simulink model "dinamica_formacao_voo"  (R2025a)
settings: Solver=ode15s  StartTime=0.0  StopTime=1424.2163  MaxStep=0.001*T  RelTol=1e-3
values from neighbouring files (symbols this model uses):
  a0 = 8e6    (= 8000000)    [main_script.m]
  controle = true    [main_script.m]
  e0 = 0.1    [main_script.m]
  f0 = 0    [main_script.m]
  i = 0    [main_script.m]
  kx = 400    [main_script.m]
  ky = 200    [main_script.m]
  kz = 200    [main_script.m]
  lambdax = 1/(1e2)    (= 0.01)    [main_script.m]
  lambday = 1/(1e2)    (= 0.01)    [main_script.m]
  lambdaz = 1/(1e2)    (= 0.01)    [main_script.m]
  mi = 3.986004418e14    (= 398600441800000)    [main_script.m]
  Omega = 0    [main_script.m]
  phix = 30    [main_script.m]
  w0 = 0    [main_script.m]
  x0_controle = -0.01127*a0    (= -90160)    [main_script.m]
  x0_real = -0.0113*a0    (= -90400)    [main_script.m]
  x_dot0 = 0.02*sqrt(mi/a0^3)*a0    [main_script.m]
  y0 = 0*a0    (= 0)    [main_script.m]
  y_dot0 = 0.02*sqrt(mi/a0^3)*a0    [main_script.m]
  z0 = 0.1*a0    (= 800000)    [main_script.m]
  z_dot0 = 0*sqrt(mi/a0^3)*a0    [main_script.m]
settings Model: Creator=Erick_Tenorio

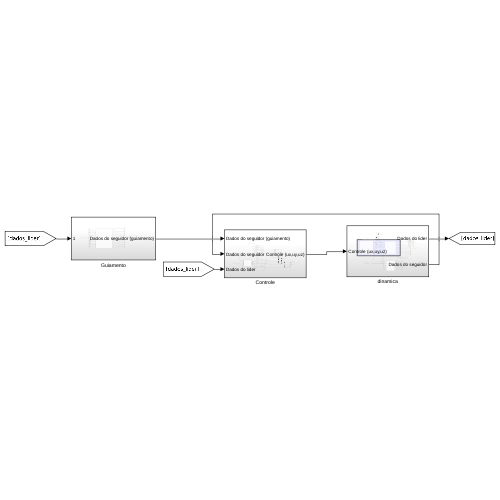
[thumbnail: Simulink's stored preview of the top-level diagram]
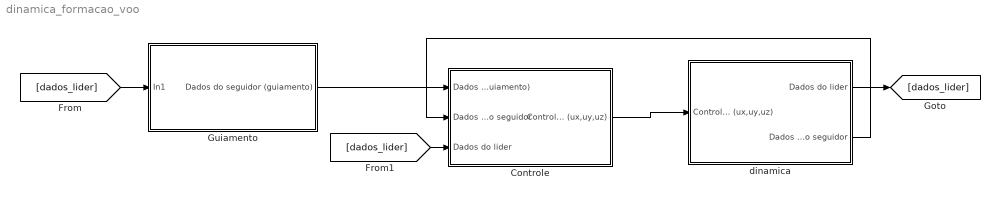
== system dinamica_formacao_voo ==
  Controle : Subsystem
  Guiamento : Subsystem
  dinamica : Subsystem
  wires:
  dinamica/1(Dados do lider) -> [dados_lider]
  [dados_lider] -> Guiamento/1(In1)
  Guiamento/1(Dados do seguidor (guiamento)) -> Controle/1(Dados do seguidor (guiamento))
  dinamica/2(Dados do seguidor) -> Controle/2(Dados do seguidor)
  [dados_lider] -> Controle/3(Dados do lider)
  Controle/1(Controle (ux,uy,uz)) -> dinamica/1(Controle (ux,uy,uz))

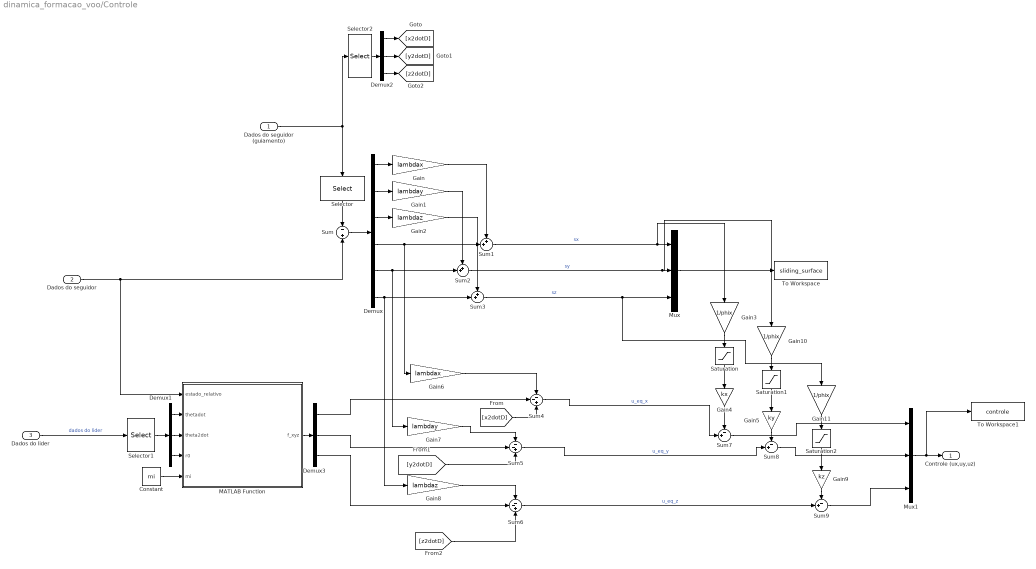
== system dinamica_formacao_voo/Controle ==
  Dados do seguidor (guiamento) : Inport
  Dados do seguidor : Inport  Port=2
  Dados do lider : Inport  Port=3
  Constant : Constant  Value=mi
  Demux : Demux  Outputs=6
  Demux1 : Demux  Outputs=3
  Demux2 : Demux  Outputs=3
  Demux3 : Demux  Outputs=3
  Gain : Gain  Gain=lambdax
  Gain1 : Gain  Gain=lambday
  Gain10 : Gain  Gain=1/phix
  Gain11 : Gain  Gain=1/phix
  Gain2 : Gain  Gain=lambdaz
  Gain3 : Gain  Gain=1/phix
  Gain4 : Gain  Gain=kx
  Gain5 : Gain  Gain=ky
  Gain6 : Gain  Gain=lambdax
  Gain7 : Gain  Gain=lambday
  Gain8 : Gain  Gain=lambdaz
  Gain9 : Gain  Gain=kz
  MATLAB Function : MATLAB Function  TreatAsAtomicUnit=on
  Mux : Mux  Inputs=3
  Mux1 : Mux  Inputs=3
  Saturation : Saturate  UpperLimit=1  LowerLimit=-1
  Saturation1 : Saturate  UpperLimit=1  LowerLimit=-1
  Saturation2 : Saturate  UpperLimit=1  LowerLimit=-1
  Selector : Selector  InputPortWidth=9  IndexOptions=Index vector (dialog)  Indices=[1 2 3 4 5 6]  OutputSizes=1
  Selector1 : Selector  InputPortWidth=7  IndexOptions=Index vector (dialog)  Indices=[3 4 1]  OutputSizes=1
  Selector2 : Selector  InputPortWidth=9  IndexOptions=Index vector (dialog)  Indices=[7 8 9]  OutputSizes=1
  Sum : Sum  Inputs=-|+
  Sum1 : Sum  Inputs=++|
  Sum2 : Sum  Inputs=++|
  Sum3 : Sum  Inputs=++|
  Sum4 : Sum  Inputs=--+
  Sum5 : Sum  Inputs=--+
  Sum6 : Sum  Inputs=--+
  Sum7 : Sum  Inputs=-+|
  Sum8 : Sum  Inputs=-+|
  Sum9 : Sum  Inputs=-+|
  To Workspace : ToWorkspace  VariableName=sliding_surface  SaveFormat=Timeseries  SampleTime=-1
  To Workspace1 : ToWorkspace  VariableName=controle  SaveFormat=Timeseries  SampleTime=-1
  Controle (ux,uy,uz) : Outport
  wires:
  Dados do seguidor (guiamento)/1 -> Selector2/1, Selector/1
  Dados do seguidor/1 -> Sum/2, MATLAB Function/1(estado_relativo)
  Sum/1 -> Demux/1
  Demux/1 -> Gain/1
  Demux/2 -> Gain1/1
  Demux/3 -> Gain2/1
  Gain/1 -> Sum1/1
  Demux/4 -> Gain6/1, Sum1/2
  Gain1/1 -> Sum2/1
  Demux/5 -> Gain7/1, Sum2/2
  Gain2/1 -> Sum3/1
  Demux/6 -> Gain8/1, Sum3/2
  Sum1/1 -> Mux/1, Gain3/1  "sx"
  Sum2/1 -> Gain10/1, Mux/2  "sy"
  Sum3/1 -> Gain11/1, Mux/3  "sz"
  Mux/1 -> To Workspace/1
  Dados do lider/1 -> Selector1/1  "dados do lider"
  Constant/1 -> MATLAB Function/5(mi)
  Selector/1 -> Sum/1
  Selector1/1 -> Demux1/1
  Demux1/1 -> MATLAB Function/2(thetadot)
  Demux1/2 -> MATLAB Function/3(theta2dot)
  Demux1/3 -> MATLAB Function/4(r0)
  Demux2/1 -> [x2dotD]
  Demux2/2 -> [y2dotD]
  Demux2/3 -> [z2dotD]
  Selector2/1 -> Demux2/1
  Gain6/1 -> Sum4/1
  Gain7/1 -> Sum5/1
  Gain8/1 -> Sum6/1
  [x2dotD] -> Sum4/3
  [y2dotD] -> Sum5/3
  [z2dotD] -> Sum6/3
  Sum5/1 -> Sum8/2  "u_eq_y"
  Sum6/1 -> Sum9/2  "u_eq_z"
  Sum4/1 -> Sum7/2  "u_eq_x"
  Gain3/1 -> Saturation/1
  Gain11/1 -> Saturation2/1
  Gain10/1 -> Saturation1/1
  Saturation/1 -> Gain4/1
  Saturation1/1 -> Gain5/1
  Saturation2/1 -> Gain9/1
  Gain9/1 -> Sum9/1
  Gain5/1 -> Sum8/1
  Gain4/1 -> Sum7/1
  Mux1/1 -> To Workspace1/1, Controle (ux,uy,uz)/1
  Sum7/1 -> Mux1/1
  Sum8/1 -> Mux1/2
  Sum9/1 -> Mux1/3
  MATLAB Function/1(f_xyz) -> Demux3/1
  Demux3/1 -> Sum4/2
  Demux3/2 -> Sum5/2
  Demux3/3 -> Sum6/2

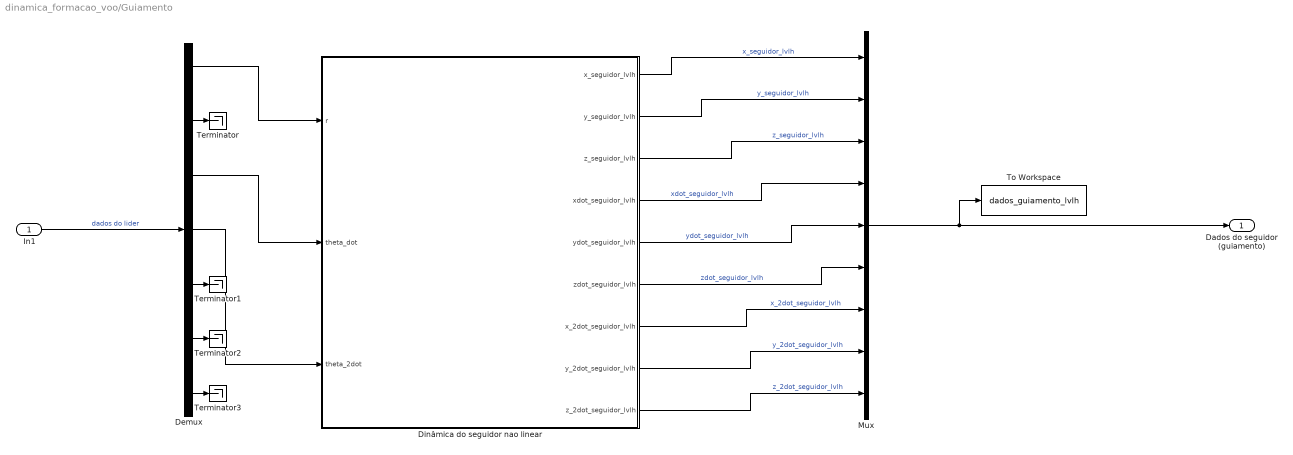
== system dinamica_formacao_voo/Guiamento ==
  In1 : Inport
  Demux : Demux  Outputs=7
  Dinâmica do seguidor nao linear : Subsystem
  Mux : Mux  Inputs=9
  Terminator{,1..3} (4 alike) : Terminator
  To Workspace : ToWorkspace  VariableName=dados_guiamento_lvlh  SaveFormat=Timeseries  SampleTime=-1
  Dados do seguidor (guiamento) : Outport
  wires:
  In1/1 -> Demux/1  "dados do lider"
  Dinâmica do seguidor nao linear/2(y_seguidor_lvlh) -> Mux/2  "y_seguidor_lvlh"
  Dinâmica do seguidor nao linear/3(z_seguidor_lvlh) -> Mux/3  "z_seguidor_lvlh"
  Dinâmica do seguidor nao linear/1(x_seguidor_lvlh) -> Mux/1  "x_seguidor_lvlh"
  Dinâmica do seguidor nao linear/4(xdot_seguidor_lvlh) -> Mux/4  "xdot_seguidor_lvlh"
  Dinâmica do seguidor nao linear/5(ydot_seguidor_lvlh) -> Mux/5  "ydot_seguidor_lvlh"
  Dinâmica do seguidor nao linear/6(zdot_seguidor_lvlh) -> Mux/6  "zdot_seguidor_lvlh"
  Mux/1 -> To Workspace/1, Dados do seguidor (guiamento)/1
  Demux/1 -> Dinâmica do seguidor nao linear/1(r)
  Demux/3 -> Dinâmica do seguidor nao linear/2(theta_dot)
  Demux/4 -> Dinâmica do seguidor nao linear/3(theta_2dot)
  Demux/2 -> Terminator/1
  Demux/5 -> Terminator1/1
  Demux/6 -> Terminator2/1
  Demux/7 -> Terminator3/1
  Dinâmica do seguidor nao linear/9(z_2dot_seguidor_lvlh) -> Mux/9  "z_2dot_seguidor_lvlh"
  Dinâmica do seguidor nao linear/8(y_2dot_seguidor_lvlh) -> Mux/8  "y_2dot_seguidor_lvlh"
  Dinâmica do seguidor nao linear/7(x_2dot_seguidor_lvlh) -> Mux/7  "x_2dot_seguidor_lvlh"

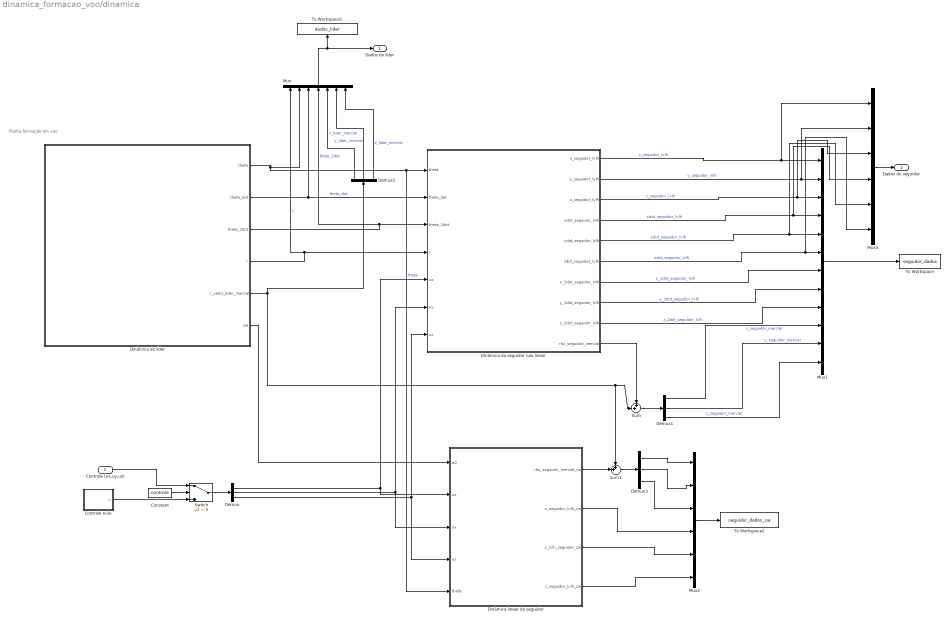
== system dinamica_formacao_voo/dinamica ==
  note: Planta formação em voo
  Controle (ux,uy,uz) : Inport
  Constant : Constant  Value=controle
  Controle nulo : Subsystem
  Demux{,1..3} (4 alike) : Demux  Outputs=3
  Dinâmica do líder : Subsystem
  Dinâmica do seguidor nao linear : Subsystem
  Dinâmica linear do seguidor : Subsystem
  Mux : Mux  Inputs=7
  Mux1 : Mux  Inputs=12
  Mux2 : Mux  Inputs=6
  Mux3 : Mux  Inputs=6
  Sum : Sum  Inputs=++|
  Sum1 : Sum  Inputs=++|
  Switch : Switch  Criteria=u2 > Threshold  SaturateOnIntegerOverflow=off  InputSameDT=off
  To Workspace : ToWorkspace  VariableName=seguidor_dados  SaveFormat=Timeseries  SampleTime=-1
  To Workspace1 : ToWorkspace  VariableName=dados_lider  SaveFormat=Timeseries  SampleTime=-1
  To Workspace2 : ToWorkspace  VariableName=seguidor_dados_cw  SaveFormat=Timeseries  SampleTime=-1
  Dados do lider : Outport
  Dados do seguidor : Outport  Port=2
  wires:
  Dinâmica do seguidor nao linear/7(x_2dot_seguidor_lvlh) -> Mux1/7  "x_2dot_seguidor_lvlh"
  Dinâmica do seguidor nao linear/10(rho_seguidor_inercial) -> Sum/1
  Demux2/3 -> Mux/7  "z_lider_inercial"
  Dinâmica do líder/5(r_vetor_lider_inercial) -> Sum1/1, Sum/2, Demux2/1
  Dinâmica do líder/6(a0) -> Dinâmica linear do seguidor/1(a0)
  Dinâmica do seguidor nao linear/5(ydot_seguidor_lvlh) -> Mux3/5, Mux1/5  "ydot_seguidor_lvlh"
  Demux1/3 -> Mux1/12  "z_seguidor_inercial"
  Demux/2 -> Dinâmica do seguidor nao linear/6(uy), Dinâmica linear do seguidor/3(uy)
  Demux3/3 -> Mux2/3
  Demux3/2 -> Mux2/2
  Demux1/2 -> Mux1/11  "y_seguidor_inercial"
  Dinâmica do seguidor nao linear/1(x_seguidor_lvlh) -> Mux3/1, Mux1/1  "x_seguidor_lvlh"
  Demux/1 -> Dinâmica do seguidor nao linear/5(ux), Dinâmica linear do seguidor/2(ux)
  Dinâmica do seguidor nao linear/9(z_2dot_seguidor_lvlh) -> Mux1/9  "z_2dot_seguidor_lvlh"
  Dinâmica do líder/3(theta_2dot) -> Mux/4, Dinâmica do seguidor nao linear/3(theta_2dot)  "theta_2dot"
  Mux/1 -> Dados do lider/1, To Workspace1/1
  Demux/3 -> Dinâmica do seguidor nao linear/7(uz), Dinâmica linear do seguidor/4(uz)
  Dinâmica do seguidor nao linear/8(y_2dot_seguidor_lvlh) -> Mux1/8  "y_2dot_seguidor_lvlh"
  Dinâmica do líder/4(r) -> Dinâmica do seguidor nao linear/4(r), Mux/1  "r"
  Dinâmica do seguidor nao linear/4(xdot_seguidor_lvlh) -> Mux3/4, Mux1/4  "xdot_seguidor_lvlh"
  Dinâmica do líder/1(theta) -> Dinâmica linear do seguidor/5(theta), Dinâmica do seguidor nao linear/1(theta), Mux/2  "theta"
  Mux1/1 -> To Workspace/1
  Demux2/1 -> Mux/5  "x_lider_inercial"
  Dinâmica do líder/2(theta_dot) -> Dinâmica do seguidor nao linear/2(theta_dot), Mux/3  "theta_dot"
  Demux2/2 -> Mux/6  "y_lider_inercial"
  Sum1/1 -> Demux3/1
  Dinâmica linear do seguidor/1(rho_seguidor_inercial_cw) -> Sum1/2
  Dinâmica do seguidor nao linear/6(zdot_seguidor_lvlh) -> Mux3/6, Mux1/6  "zdot_seguidor_lvlh"
  Dinâmica do seguidor nao linear/3(z_seguidor_lvlh) -> Mux3/3, Mux1/3  "z_seguidor_lvlh"
  Dinâmica do seguidor nao linear/2(y_seguidor_lvlh) -> Mux3/2, Mux1/2  "y_seguidor_lvlh"
  Sum/1 -> Demux1/1
  Demux1/1 -> Mux1/10  "x_seguidor_inercial"
  Dinâmica linear do seguidor/3(y_lvlh_seguidor_cw) -> Mux2/5
  Mux2/1 -> To Workspace2/1
  Dinâmica linear do seguidor/2(x_seguidor_lvlh_cw) -> Mux2/4
  Dinâmica linear do seguidor/4(z_seguidor_lvlh_cw) -> Mux2/6
  Demux3/1 -> Mux2/1
  Controle (ux,uy,uz)/1 -> Switch/1
  Controle nulo/1(u) -> Switch/3
  Switch/1 -> Demux/1
  Constant/1 -> Switch/2
  Mux3/1 -> Dados do seguidor/1

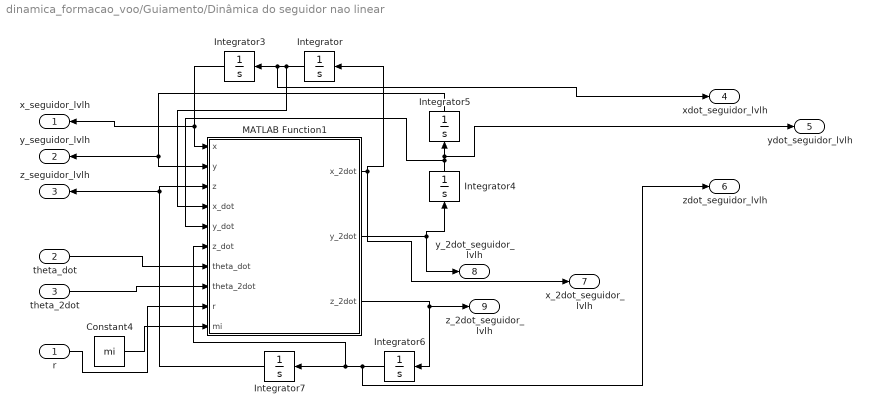
== system dinamica_formacao_voo/Guiamento/Dinâmica do seguidor nao linear ==
  r : Inport
  theta_dot : Inport  Port=2
  theta_2dot : Inport  Port=3
  Constant4 : Constant  Value=mi
  Integrator : Integrator  InitialCondition=x_dot0
  Integrator3 : Integrator  InitialCondition=x0_controle
  Integrator4 : Integrator  InitialCondition=y_dot0
  Integrator5 : Integrator  InitialCondition=y0
  Integrator6 : Integrator  InitialCondition=z_dot0
  Integrator7 : Integrator  InitialCondition=z0
  MATLAB Function1 : MATLAB Function  TreatAsAtomicUnit=on
  x_seguidor_lvlh : Outport
  y_seguidor_lvlh : Outport  Port=2
  z_seguidor_lvlh : Outport  Port=3
  xdot_seguidor_lvlh : Outport  Port=4
  ydot_seguidor_lvlh : Outport  Port=5
  zdot_seguidor_lvlh : Outport  Port=6
  x_2dot_seguidor_lvlh : Outport  Port=7
  y_2dot_seguidor_lvlh : Outport  Port=8
  z_2dot_seguidor_lvlh : Outport  Port=9
  wires:
  Integrator6/1 -> zdot_seguidor_lvlh/1, MATLAB Function1/6(z_dot), Integrator7/1
  Integrator/1 -> MATLAB Function1/4(x_dot), xdot_seguidor_lvlh/1, Integrator3/1
  MATLAB Function1/2(y_2dot) -> Integrator4/1, y_2dot_seguidor_lvlh/1
  Integrator5/1 -> MATLAB Function1/2(y), y_seguidor_lvlh/1
  MATLAB Function1/3(z_2dot) -> Integrator6/1, z_2dot_seguidor_lvlh/1
  Integrator3/1 -> MATLAB Function1/1(x), x_seguidor_lvlh/1
  Integrator4/1 -> MATLAB Function1/5(y_dot), ydot_seguidor_lvlh/1, Integrator5/1
  theta_dot/1 -> MATLAB Function1/7(theta_dot)
  Constant4/1 -> MATLAB Function1/10(mi)
  theta_2dot/1 -> MATLAB Function1/8(theta_2dot)
  MATLAB Function1/1(x_2dot) -> Integrator/1, x_2dot_seguidor_lvlh/1
  Integrator7/1 -> z_seguidor_lvlh/1, MATLAB Function1/3(z)
  r/1 -> MATLAB Function1/9(r)

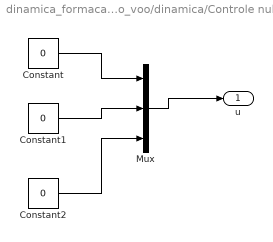
== system dinamica_formacao_voo/dinamica/Controle nulo ==
  Constant : Constant  Value=0
  Constant1 : Constant  Value=0
  Constant2 : Constant  Value=0
  Mux : Mux  Inputs=3
  u : Outport
  wires:
  Constant/1 -> Mux/1
  Constant1/1 -> Mux/2
  Constant2/1 -> Mux/3
  Mux/1 -> u/1

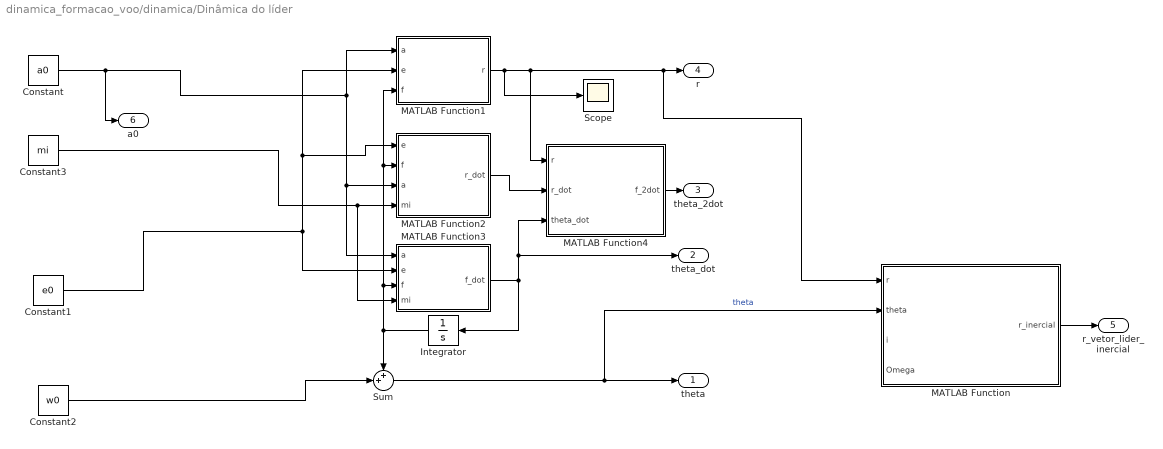
== system dinamica_formacao_voo/dinamica/Dinâmica do líder ==
  Constant : Constant  Value=a0
  Constant1 : Constant  Value=e0
  Constant2 : Constant  Value=w0
  Constant3 : Constant  Value=mi
  Integrator : Integrator  InitialCondition=f0
  MATLAB Function : MATLAB Function  TreatAsAtomicUnit=on
  MATLAB Function1 : MATLAB Function  TreatAsAtomicUnit=on
  MATLAB Function2 : MATLAB Function  TreatAsAtomicUnit=on
  MATLAB Function3 : MATLAB Function  TreatAsAtomicUnit=on
  MATLAB Function4 : MATLAB Function  TreatAsAtomicUnit=on
  Scope : Scope
      settings: ActiveDisplayYMinimum=7.0E+6  ActiveDisplayYMaximum=9.0E+6
  Sum : Sum  Inputs=++|
  theta : Outport
  theta_dot : Outport  Port=2
  theta_2dot : Outport  Port=3
  r : Outport  Port=4
  r_vetor_lider_inercial : Outport  Port=5
  a0 : Outport  Port=6
  wires:
  Constant/1 -> a0/1, MATLAB Function3/1(a), MATLAB Function2/3(a), MATLAB Function1/1(a)
  Constant1/1 -> MATLAB Function2/1(e), MATLAB Function1/2(e), MATLAB Function3/2(e)
  Constant2/1 -> Sum/2
  Constant3/1 -> MATLAB Function3/4(mi), MATLAB Function2/4(mi)
  MATLAB Function3/1(f_dot) -> theta_dot/1, MATLAB Function4/3(theta_dot), Integrator/1
  MATLAB Function1/1(r) -> Scope/1, MATLAB Function/1(r), r/1, MATLAB Function4/1(r)
  Integrator/1 -> Sum/1, MATLAB Function1/3(f), MATLAB Function2/2(f), MATLAB Function3/3(f)
  Sum/1 -> MATLAB Function/2(theta), theta/1  "theta"
  MATLAB Function2/1(r_dot) -> MATLAB Function4/2(r_dot)
  MATLAB Function4/1(f_2dot) -> theta_2dot/1
  MATLAB Function/1(r_inercial) -> r_vetor_lider_inercial/1

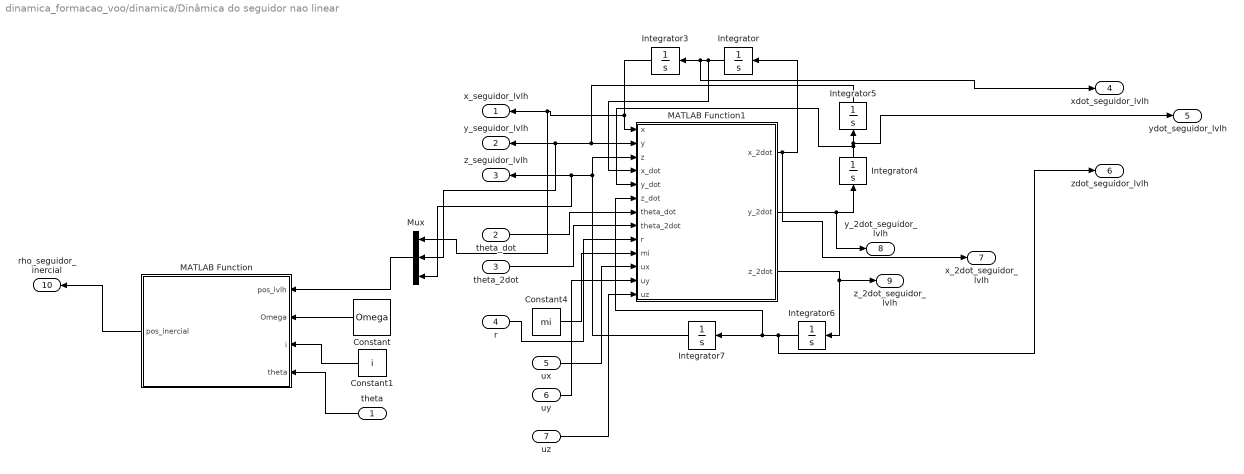
== system dinamica_formacao_voo/dinamica/Dinâmica do seguidor nao linear ==
  theta : Inport
  theta_dot : Inport  Port=2
  theta_2dot : Inport  Port=3
  r : Inport  Port=4
  ux : Inport  Port=5
  uy : Inport  Port=6
  uz : Inport  Port=7
  Constant : Constant  Value=Omega
  Constant1 : Constant  Value=i
  Constant4 : Constant  Value=mi
  Integrator : Integrator  InitialCondition=x_dot0
  Integrator3 : Integrator  InitialCondition=x0_real
  Integrator4 : Integrator  InitialCondition=y_dot0
  Integrator5 : Integrator  InitialCondition=y0
  Integrator6 : Integrator  InitialCondition=z_dot0
  Integrator7 : Integrator  InitialCondition=z0
  MATLAB Function : MATLAB Function  TreatAsAtomicUnit=on
  MATLAB Function1 : MATLAB Function  TreatAsAtomicUnit=on
  Mux : Mux  Inputs=3
  x_seguidor_lvlh : Outport
  y_seguidor_lvlh : Outport  Port=2
  z_seguidor_lvlh : Outport  Port=3
  xdot_seguidor_lvlh : Outport  Port=4
  ydot_seguidor_lvlh : Outport  Port=5
  zdot_seguidor_lvlh : Outport  Port=6
  x_2dot_seguidor_lvlh : Outport  Port=7
  y_2dot_seguidor_lvlh : Outport  Port=8
  z_2dot_seguidor_lvlh : Outport  Port=9
  rho_seguidor_inercial : Outport  Port=10
  wires:
  Integrator6/1 -> zdot_seguidor_lvlh/1, MATLAB Function1/6(z_dot), Integrator7/1
  Integrator/1 -> MATLAB Function1/4(x_dot), xdot_seguidor_lvlh/1, Integrator3/1
  MATLAB Function1/2(y_2dot) -> y_2dot_seguidor_lvlh/1, Integrator4/1
  Integrator5/1 -> MATLAB Function1/2(y), Mux/2, y_seguidor_lvlh/1
  MATLAB Function1/3(z_2dot) -> Integrator6/1, z_2dot_seguidor_lvlh/1
  Integrator3/1 -> MATLAB Function1/1(x), x_seguidor_lvlh/1, Mux/1
  Integrator4/1 -> MATLAB Function1/5(y_dot), ydot_seguidor_lvlh/1, Integrator5/1
  theta_dot/1 -> MATLAB Function1/7(theta_dot)
  Constant4/1 -> MATLAB Function1/10(mi)
  theta_2dot/1 -> MATLAB Function1/8(theta_2dot)
  MATLAB Function1/1(x_2dot) -> x_2dot_seguidor_lvlh/1, Integrator/1
  Integrator7/1 -> Mux/3, z_seguidor_lvlh/1, MATLAB Function1/3(z)
  r/1 -> MATLAB Function1/9(r)
  ux/1 -> MATLAB Function1/11(ux)
  uy/1 -> MATLAB Function1/12(uy)
  uz/1 -> MATLAB Function1/13(uz)
  Mux/1 -> MATLAB Function/1(pos_lvlh)
  Constant/1 -> MATLAB Function/2(Omega)
  Constant1/1 -> MATLAB Function/3(i)
  theta/1 -> MATLAB Function/4(theta)
  MATLAB Function/1(pos_inercial) -> rho_seguidor_inercial/1

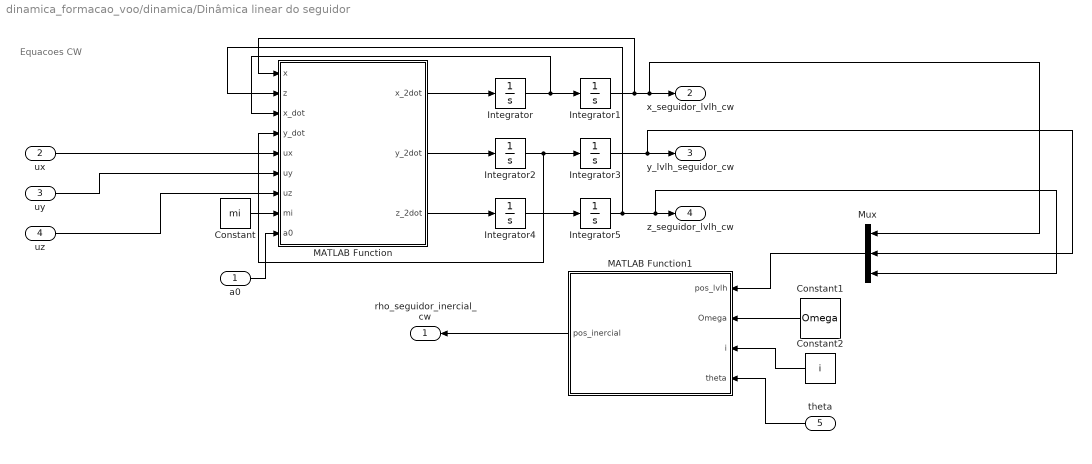
== system dinamica_formacao_voo/dinamica/Dinâmica linear do seguidor ==
  note: Equacoes CW
  a0 : Inport
  ux : Inport  Port=2
  uy : Inport  Port=3
  uz : Inport  Port=4
  theta : Inport  Port=5
  Constant : Constant  Value=mi
  Constant1 : Constant  Value=Omega
  Constant2 : Constant  Value=i
  Integrator : Integrator  InitialCondition=x_dot0
  Integrator1 : Integrator  InitialCondition=x0_real
  Integrator2 : Integrator  InitialCondition=y_dot0
  Integrator3 : Integrator  InitialCondition=y0
  Integrator4 : Integrator  InitialCondition=z_dot0
  Integrator5 : Integrator  InitialCondition=z0
  MATLAB Function : MATLAB Function  TreatAsAtomicUnit=on
  MATLAB Function1 : MATLAB Function  TreatAsAtomicUnit=on
  Mux : Mux  Inputs=3
  rho_seguidor_inercial_cw : Outport
  x_seguidor_lvlh_cw : Outport  Port=2
  y_lvlh_seguidor_cw : Outport  Port=3
  z_seguidor_lvlh_cw : Outport  Port=4
  wires:
  MATLAB Function/1(x_2dot) -> Integrator/1
  Integrator/1 -> MATLAB Function/3(x_dot), Integrator1/1
  MATLAB Function/2(y_2dot) -> Integrator2/1
  Integrator2/1 -> MATLAB Function/4(y_dot), Integrator3/1
  MATLAB Function/3(z_2dot) -> Integrator4/1
  Integrator4/1 -> Integrator5/1
  Constant/1 -> MATLAB Function/8(mi)
  a0/1 -> MATLAB Function/9(a0)
  uz/1 -> MATLAB Function/7(uz)
  uy/1 -> MATLAB Function/6(uy)
  ux/1 -> MATLAB Function/5(ux)
  Mux/1 -> MATLAB Function1/1(pos_lvlh)
  Integrator5/1 -> Mux/3, z_seguidor_lvlh_cw/1, MATLAB Function/2(z)
  Integrator1/1 -> Mux/1, x_seguidor_lvlh_cw/1, MATLAB Function/1(x)
  MATLAB Function1/1(pos_inercial) -> rho_seguidor_inercial_cw/1
  Constant1/1 -> MATLAB Function1/2(Omega)
  Constant2/1 -> MATLAB Function1/3(i)
  Integrator3/1 -> Mux/2, y_lvlh_seguidor_cw/1
  theta/1 -> MATLAB Function1/4(theta)

== matlab function dinamica_formacao_voo/dinamica/Dinâmica linear do seguidor/MATLAB Function ==
  data: x input; z input; x_dot input; y_dot input; x_2dot output; ux input; uy input; uz input; mi input; a0 input; y_2dot output; z_2dot output
function [x_2dot, y_2dot, z_2dot] = calcular_aceleracao_cw(x,z,x_dot,y_dot, ux,uy,uz,mi, a0)
% calcular_aceleracao_cw: Calcula a aceleração relativa [ẍ; ÿ; ż] de um
% seguidor com base nas equações de Clohessy-Wiltshire (CW) forçadas.
%
% A implementação é baseada nas Equações 5.7, 5.8 e 5.9 do livro
% "Spacecraft Formation Flying" por Alfriend et al.
%
% ENTRADAS:
%   estado_relativo - Vetor coluna 6x1 com o estado relativo atual:
%                     [x; y; z; x_dot; y_dot; z_dot] em [km] e [km/s].
%   u_controle      - Vetor coluna 3x1 com as acelerações de controle
%                     aplicadas [ux; uy; uz] em [km/s^2].
%   a0              - Escalar. O semieixo maior da órbita do líder [km].
%
% SAÍDA:
%   aceleracao_relativa - Vetor coluna 3x1 com as acelerações resultantes
%                         [ẍ; ÿ; ż] em [km/s^2].

% --- 1. Constantes e Parâmetros Orbitais ---
% Parâmetro gravitacional da Terra

% Calcula o movimento médio 'n' da órbita do líder
n = sqrt(mi / a0^3); % rad/s



% z_dot não é usado nas equações CW de aceleração

% --- 3. Cálculo das Acelerações (rearranjando as equações CW) ---
% De eq. 5.7: x_2dot = 3*n^2*x + 2*n*y_dot + ux
x_2dot = 3 * n^2 * x + 2 * n * y_dot + ux;

% De eq. 5.8: y_2dot = -2*n*x_dot + uy
y_2dot = -2 * n * x_dot + uy;

% De eq. 5.9: z_2dot = -n^2*z + uz
z_2dot = -n^2 * z + uz;



end

== matlab function dinamica_formacao_voo/dinamica/Dinâmica linear do seguidor/MATLAB Function1 ==
  data: pos_lvlh input; Omega input; pos_inercial output; i input; theta input
function pos_inercial = lvlh_para_inercial(pos_lvlh, Omega, i, theta)
% lvlh_para_inercial: Transforma um vetor posição do sistema LVLH do líder
% para o sistema de referência inercial (ECI).
%
% A matriz de transformação é a transposta da matriz T_I^L da 
% Equação 4.100 do livro "Spacecraft Formation Flying" por Alfriend et al.
%
% ENTRADAS:
%   pos_lvlh   - Vetor posição 3x1 [x; y; z] no sistema LVLH [km].
%   Omega      - Ascensão Reta do Nodo Ascendente (RAAN) do líder [rad].
%   i          - Inclinação da órbita do líder [rad].
%   theta      - Argumento de Latitude (theta = omega + f) do líder [rad].
%
% SAÍDA:
%   pos_inercial - Vetor posição 3x1 [X; Y; Z] no sistema inercial [km].

% Calcula os senos e cossenos para facilitar a leitura
c_O = cos(Omega);
s_O = sin(Omega);
c_i = cos(i);
s_i = sin(i);
c_t = cos(theta);
s_t = sin(theta);

% Monta a matriz T_IL (T que transforma de Inercial para LVLH)
% conforme a Equação 4.100
T_IL = [ c_O*c_t - s_O*s_t*c_i,   s_O*c_t + c_O*s_t*c_i,  s_t*s_i;
        -c_O*s_t - s_O*c_t*c_i,  -s_O*s_t + c_O*c_t*c_i,  c_t*s_i;
         s_O*s_i,                 -c_O*s_i,                 c_i      ];

% A transformação de LVLH para Inercial usa a transposta de T_IL
T_LI = T_IL';

% Realiza a transformação
pos_inercial = T_LI * pos_lvlh;

end

== matlab function dinamica_formacao_voo/Controle/MATLAB Function ==
  data: estado_relativo input size=[6,1]; f_xyz output size=[3,1]; thetadot input; theta2dot input; r0 input; mi input
function f_xyz = calcular_dinamica_naolinear_f(estado_relativo, thetadot, theta2dot, r0, mi)
% calcular_dinamica_naolinear_f: Calcula a parte não linear f(x) da
% dinâmica relativa do satélite (ẍ = f(x) + u).
%
% A implementação é baseada nas equações não lineares do movimento
% relativo no referencial LVLH, conforme as Equações 4.14-4.16 do livro
% "Spacecraft Formation Flying" por Alfriend et al.
%
% ENTRADAS:
%   estado_relativo - Vetor coluna 6x1 com o estado relativo atual:
%                     [x; y; z; xdot; ydot; zdot] em [km] e [km/s].
%   thetadot        - Velocidade angular do líder (d(f0)/dt) [rad/s].
%   theta2dot       - Aceleração angular do líder (d^2(f0)/dt^2) [rad/s^2].
%   r0              - Raio escalar (magnitude da posição) do líder [km].
%   mi              - Parâmetro gravitacional padrão do corpo central [km^3/s^2].
%
% SAÍDA:
%   f_xyz           - Vetor coluna 3x1 com os termos da dinâmica não linear
%                     [fx; fy; fz] em [km/s^2].

% --- 1. Extração dos Estados ---
x = estado_relativo(1);
y = estado_relativo(2);
z = estado_relativo(3);
xdot = estado_relativo(4);
ydot = estado_relativo(5);
% zdot não aparece nos termos de f(x)

% --- 2. Cálculo de Termos Comuns ---
pos_seguidor_inercial_mag_cubed = ((r0 + x)^2 + y^2 + z^2)^(3/2);

% --- 3. Cálculo dos Componentes de f(x) ---

% Componente fx
fx = 2*thetadot*ydot + theta2dot*y + thetadot^2*x ...
     - mi*(r0 + x)/pos_seguidor_inercial_mag_cubed + mi/r0^2;

% Componente fy
fy = -2*thetadot*xdot - theta2dot*x + thetadot^2*y ...
     - mi*y/pos_seguidor_inercial_mag_cubed;

% Componente fz
fz = -mi*z/pos_seguidor_inercial_mag_cubed;

% --- 4. Monta o Vetor de Saída ---
f_xyz = [fx; fy; fz];

end

== matlab function dinamica_formacao_voo/Guiamento/Dinâmica do seguidor nao linear/MATLAB Function1 ==
  data: x input; x_2dot output; y input; z input; x_dot input; y_dot input; z_dot input; theta_dot input; theta_2dot input; r input; mi input; y_2dot output; z_2dot output
function [x_2dot,y_2dot,z_2dot] = f_rel_seguidor(x,y,z,x_dot,y_dot,z_dot,theta_dot,theta_2dot,r,mi)

x_2dot = 2*theta_dot*y_dot + theta_2dot*y + (theta_dot^2)*x ...
          - ((mi*(r + x))/((r + x)^2 + y^2 + z^2)^(3/2)) + (mi/r^2);

y_2dot = -2*theta_dot*x_dot - theta_2dot*x + (theta_dot^2)*y ...
          - ((mi*y)/((r + x)^2 + y^2 + z^2)^(3/2));  

z_2dot = - ((mi*z)/((r + x)^2 + y^2 + z^2)^(3/2));

end

== matlab function dinamica_formacao_voo/dinamica/Dinâmica do líder/MATLAB Function1 ==
  data: a input; r output; e input; f input
function r = leader_r(a,e,f)
r = (a*(1-e^2))/(1+e*cos(f));
end

== matlab function dinamica_formacao_voo/dinamica/Dinâmica do seguidor nao linear/MATLAB Function ==
  data: pos_lvlh input; Omega input; pos_inercial output; i input; theta input
function pos_inercial = lvlh_para_inercial(pos_lvlh, Omega, i, theta)
% lvlh_para_inercial: Transforma um vetor posição do sistema LVLH do líder
% para o sistema de referência inercial (ECI).
%
% A matriz de transformação é a transposta da matriz T_I^L da 
% Equação 4.100 do livro "Spacecraft Formation Flying" por Alfriend et al.
%
% ENTRADAS:
%   pos_lvlh   - Vetor posição 3x1 [x; y; z] no sistema LVLH [km].
%   Omega      - Ascensão Reta do Nodo Ascendente (RAAN) do líder [rad].
%   i          - Inclinação da órbita do líder [rad].
%   theta      - Argumento de Latitude (theta = omega + f) do líder [rad].
%
% SAÍDA:
%   pos_inercial - Vetor posição 3x1 [X; Y; Z] no sistema inercial [km].

% Calcula os senos e cossenos para facilitar a leitura
c_O = cos(Omega);
s_O = sin(Omega);
c_i = cos(i);
s_i = sin(i);
c_t = cos(theta);
s_t = sin(theta);

% Monta a matriz T_IL (T que transforma de Inercial para LVLH)
% conforme a Equação 4.100
T_IL = [ c_O*c_t - s_O*s_t*c_i,   s_O*c_t + c_O*s_t*c_i,  s_t*s_i;
        -c_O*s_t - s_O*c_t*c_i,  -s_O*s_t + c_O*c_t*c_i,  c_t*s_i;
         s_O*s_i,                 -c_O*s_i,                 c_i      ];

% A transformação de LVLH para Inercial usa a transposta de T_IL
T_LI = T_IL';

% Realiza a transformação
pos_inercial = T_LI * pos_lvlh;

end

== matlab function dinamica_formacao_voo/dinamica/Dinâmica do líder/MATLAB Function2 ==
  data: e input; r_dot output; f input; a input; mi input
function r_dot = leader_rdot(e,f,a,mi)

r_dot = e*sin(f)*sqrt(mi/(a*(1-e^2)));
end

== matlab function dinamica_formacao_voo/dinamica/Dinâmica do líder/MATLAB Function3 ==
  data: a input; f_dot output; e input; f input; mi input
function f_dot = leader_f_dot(a,e,f,mi) % f -> anomalia verdadeira

f_dot = (sqrt(mi/(a*(1-e^2))^3))*(1+e*cos(f))^2;

end

== matlab function dinamica_formacao_voo/dinamica/Dinâmica do líder/MATLAB Function4 ==
  data: r input; f_2dot output; r_dot input; theta_dot input
function f_2dot = leader_f_2dot(r,r_dot,theta_dot)
f_2dot = -(2*r_dot*theta_dot)/r;
end

== matlab function dinamica_formacao_voo/dinamica/Dinâmica do seguidor nao linear/MATLAB Function1 ==
  data: x input; x_2dot output; y input; z input; x_dot input; y_dot input; z_dot input; theta_dot input; theta_2dot input; r input; mi input; y_2dot output; z_2dot output; ux input; uy input; uz input
function [x_2dot,y_2dot,z_2dot] = f_rel_seguidor(x,y,z,x_dot,y_dot,z_dot,theta_dot,theta_2dot,r,mi,ux,uy,uz)

x_2dot = 2*theta_dot*y_dot + theta_2dot*y + (theta_dot^2)*x ...
          - ((mi*(r + x))/((r + x)^2 + y^2 + z^2)^(3/2)) + (mi/r^2) + ux;
y_2dot = -2*theta_dot*x_dot - theta_2dot*x + (theta_dot^2)*y ...
          - ((mi*y)/((r + x)^2 + y^2 + z^2)^(3/2)) + uy;  
z_2dot = - ((mi*z)/((r + x)^2 + y^2 + z^2)^(3/2)) + uz;

end

== matlab function dinamica_formacao_voo/dinamica/Dinâmica do líder/MATLAB Function ==
  data: r input; r_inercial output; theta input; i input; Omega input
function r_inercial = perifocal_para_inercial(r, theta, i, Omega)
% perifocal_para_inercial: Transforma um vetor posição do sistema perifocal 
% para o sistema de referência inercial (ECI).
%
% A implementação é baseada na Equação 2.40 do livro "Spacecraft 
% Formation Flying" por Alfriend et al. [cite: 264]
%
% ENTRADAS:
%   r          - Raio escalar (magnitude do vetor posição) [km]
%   theta      - Argumento de latitude (theta = omega + f) [rad]
%   i          - Inclinação da órbita [rad]
%   Omega      - Ascensão Reta do Nodo Ascendente (RAAN) [rad]
%
% SAÍDA:
%   r_inercial - Vetor posição [x; y; z] no sistema inercial [km]

% Calcula os senos e cossenos para simplificar as equações
c_t = cos(theta);
s_t = sin(theta);

c_i = cos(i);
s_i = sin(i);

c_O = cos(Omega);
s_O = sin(Omega);

% Calcula as componentes do vetor inercial conforme a Equação 2.40
% Nota: O termo a(1-e^2)/(1+e*cos(f)) da equação é exatamente 'r'.
x = r * (c_t * c_O - c_i * s_t * s_O);
y = r * (c_i * c_O * s_t + c_t * s_O);
z = r * (s_i * s_t);

% Monta o vetor de saída
r_inercial = [x; y; z];

end
